simulink model "test20230615"  (R2023b)
settings: Solver=FixedStepAuto  StartTime=0.0  StopTime=20  FixedStep=0.001  RelTol=1e-3
undefined symbols (not defined in the file): DiscIntNeverNeededParam
libraries: simulink x1
settings Model: Creator=DONGGUIYI  LastModifiedBy=dgy92
settings OptimizationCC: ReuseModelBlockBuffer=off

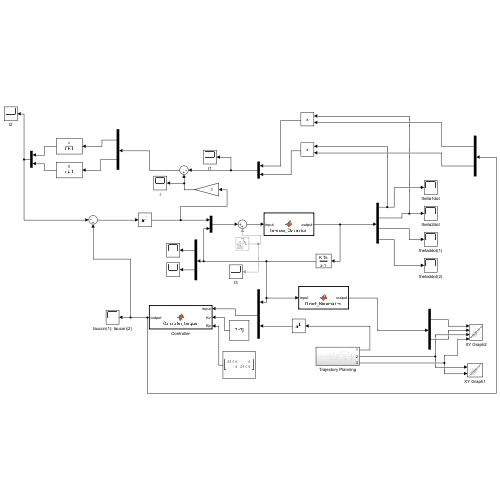
[thumbnail: Simulink's stored preview of the top-level diagram]
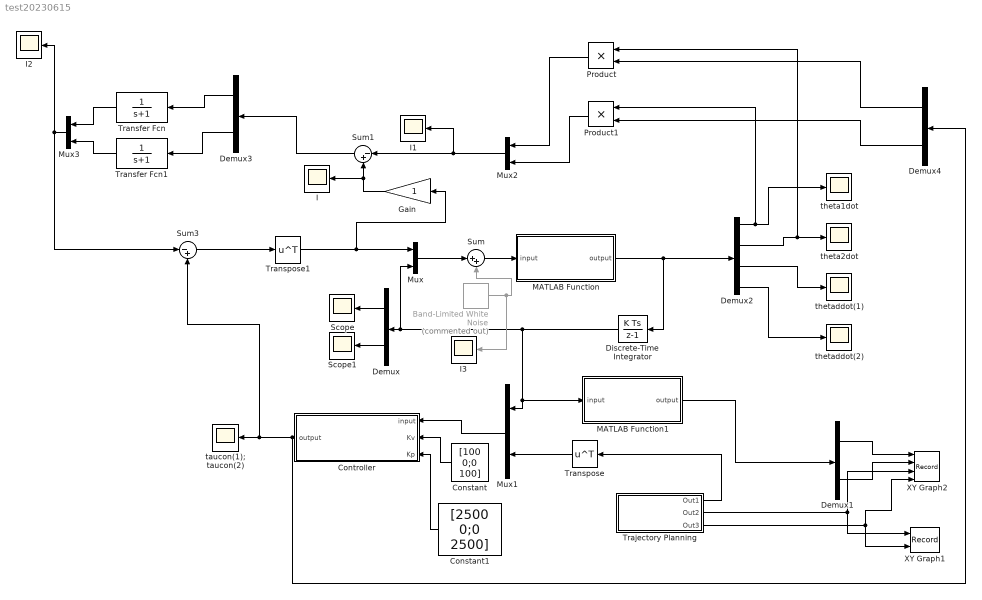
== system test20230615 ==
  Band-Limited White Noise : simulink/Sources/Band-Limited White Noise  Commented=on  Cov=[0.001]  Ts=0.1  seed=[23341]
  Constant : Constant  Value=[100 0;0 100]
  Constant1 : Constant  Value=[2500 0;0 2500]
  Controller : MATLAB Function  Tag=comp_torque  TreatAsAtomicUnit=on
  Demux{,1,3..4} (4 alike) : Demux  Outputs=2
  Demux2 : Demux
  Discrete-Time Integrator : DiscreteIntegrator  SampleTime=-1  ICPrevOutput=DiscIntNeverNeededParam  ICPrevScaledInput=DiscIntNeverNeededParam
  Gain : Gain
  I{,1..3} (4 alike) : Scope
  MATLAB Function : MATLAB Function  TreatAsAtomicUnit=on
  MATLAB Function1 : MATLAB Function  TreatAsAtomicUnit=on
  Mux : Mux  Inputs=[2,4]
  Mux1 : Mux  Inputs=2
  Mux2 : Mux  Inputs=[1,1]
  Mux3 : Mux  Inputs=[1,1]
  Product : Product
  Product1 : Product
  Scope : Scope
  Scope1 : Scope
  Sum : Sum  Inputs=|++
  Sum1 : Sum  Inputs=|-+
  Sum3 : Sum  Inputs=|-+
  Trajectory Planning : Subsystem
  Transfer Fcn : TransferFcn  Denominator=[1 1]
  Transfer Fcn1 : TransferFcn  Denominator=[1 1]
  Transpose : Math  Operator=transpose
  Transpose1 : Math  Operator=transpose
  XY Graph1 : Record  FileSettingsInternal="{\"entries\":[{\"content\":{\"excelSettings\":{\"content\":{},\"type\":\"Streamout.ExcelSettings\"}},\"type\":\"Streamout.FileSettingStorage\",\"uuid\":\"\"}],\"packageUris\":[\"http:\\/\\/schema.mathworks.com\\/mf0\\/streamout_blocks\\/R2020a\"],\"version\":\"1.0\"}"  Layout=[1 1]  SignalsInternal="{\"entries\":[{\"content\":{\"signals\":[{\"content\":{\"blockPath\":[],\"dimensions\":[1,1],\"domain\":\"\",\"lineColor\":\"#77ac30\",\"plots\":[1],\"port\":1,\"sid\":[\"\"],\"signalID\":896,\"signalName\":\"Trajectory Planning:2\"},\"type\":\"RecordBlkView.Signal\",\"uuid\":\"\"},{\"content\":{\"blockPath\":[],\"dimensions\":[1,1],\"domain\":\"\",\"lineColor\":\"#4dbeee\",\"plots\":[1],\"port\":2,\"sid\":[\"\"],\"signalID\":900,\"signalName\":\"Trajectory Planning:3\"},\"type\":\"RecordBlkView.Signal\",\"uuid\":\"\"}]},\"type\":\"RecordBlkView.InputSignals\",\"uuid\":\"\"}],\"packageUris\":[\"http:\\/\\/schema.mathworks.com\\/mf0\\/streamout_blocks\\/R2020a\"],\"version\":\"1.0\"}"  VisualizationBindings="{\"xyplotplugin\":{\"info\":[{\"series\":[{\"bindingParametersList\":[{\"parameter\":\"X-Axis\",\"signalID\":896,\"signalName\":\"Trajectory Planning:2\"},{\"parameter\":\"Y-Axis\",\"signalID\":900,\"signalName\":\"Trajectory Planning:3\"}],\"seriesID\":3912}],\"subplotID\":1}]}}"  CompatibilityTag=XY
  XY Graph2 : Record  FileSettingsInternal="{\"entries\":[{\"content\":{\"excelSettings\":{\"content\":{},\"type\":\"Streamout.ExcelSettings\"}},\"type\":\"Streamout.FileSettingStorage\",\"uuid\":\"\"}],\"packageUris\":[\"http:\\/\\/schema.mathworks.com\\/mf0\\/streamout_blocks\\/R2020a\"],\"version\":\"1.0\"}"  Layout=[1 1]  SignalsInternal="{\"entries\":[{\"content\":{\"signals\":[{\"content\":{\"blockPath\":[],\"dimensions\":[1,1],\"domain\":\"\",\"lineColor\":\"#a2142f\",\"plots\":[1],\"port\":1,\"sid\":[\"\"],\"signalID\":904,\"signalName\":\"Demux1:1\"},\"type\":\"RecordBlkView.Signal\",\"uuid\":\"\"},{\"content\":{\"blockPath\":[],\"dimensions\":[1,1],\"domain\":\"\",\"lineColor\":\"#139fff\",\"plots\":[1],\"port\":2,\"sid\":[\"\"],\"signalID\":908,\"signalName\":\"Demux1:2\"},\"type\":\"RecordBlkView.Signal\",\"uuid\":\"\"},{\"content\":{\"blockPath\":[],\"dimensions\":[1,1],\"domain\":\"\",\"lineColor\":\"#ff6929\",\"plots\":[1],\"port\":3,\"sid\":[\"\"],\"signalID\":912,\"signalName\":\"Trajectory Planning:2\"},\"type\":\"RecordBlkView.Signal\",\"uuid\":\"\"},{\"content\":{\"blockPath\":[],\"dimensions\":[1,1],\"domain\":\"\",\"lineColor\":\"#b746ff\",\"plots\":[1],\"port\":4,\"sid\":[\"\"],\"signalID\":916,\"signalName\":\"Trajectory Planning:3\"},\"type\":\"RecordBlkView.Signal\",\"uuid\":\"\"}]},\"type\":\"RecordBlkView.InputSignals\",\"uuid\":\"\"}],\"packageUris\":[\"http:\\/\\/schema.mathworks.com\\/mf0\\/streamout_blocks\\/R2020a\"],\"version\":\"1.0\"}"  VisualizationBindings="{\"xyplotplugin\":{\"info\":[{\"series\":[{\"bindingParametersList\":[{\"parameter\":\"X-Axis\",\"signalID\":904,\"signalName\":\"Demux1:1\"},{\"parameter\":\"Y-Axis\",\"signalID\":908,\"signalName\":\"Demux1:2\"}],\"seriesID\":2340},{\"bindingParametersList\":[{\"parameter\":\"X-Axis\",\"signalID\":912,\"signalName\":\"Trajectory Planning:2\"},{\"parameter\":\"Y-Axis\",\"signalID\":916,\"signalName\":\"Trajectory Planning:3\"}],\"seriesID\":45430}],\"subplotID\":1}]}}"  CompatibilityTag=XY  st=-1
  taucon(1); taucon(2) : Scope
  theta1dot : Scope
  theta2dot : Scope
  thetaddot(1) : Scope
  thetaddot(2) : Scope
  wires:
  Discrete-Time Integrator/1 -> Mux1/1, MATLAB Function1/1(input), Mux/2, Demux/1
  Demux/2 -> Scope1/1
  Demux/1 -> Scope/1
  MATLAB Function1/1(output) -> Demux1/1
  Demux1/1 -> XY Graph2/1
  Demux1/2 -> XY Graph2/2
  Transpose/1 -> Mux1/2
  Trajectory Planning/1(Out1) -> Transpose/1
  Controller/1(output) -> Demux4/1, Sum3/2, taucon(1); taucon(2)/1
  Mux1/1 -> Controller/1(input)
  Trajectory Planning/2(Out2) -> XY Graph2/3, XY Graph1/1
  Trajectory Planning/3(Out3) -> XY Graph2/4, XY Graph1/2
  Constant/1 -> Controller/2(Kv)
  Constant1/1 -> Controller/3(Kp)
  Demux2/4 -> thetaddot(2)/1
  Demux2/3 -> thetaddot(1)/1
  Demux2/2 -> Product/1, theta2dot/1
  Demux2/1 -> Product1/1, theta1dot/1
  Band-Limited White Noise/1 -> I3/1, Sum/2
  MATLAB Function/1(output) -> Discrete-Time Integrator/1, Demux2/1
  Sum/1 -> MATLAB Function/1(input)
  Mux/1 -> Sum/1
  Mux2/1 -> I1/1, Sum1/1
  Gain/1 -> I/1, Sum1/2
  Sum3/1 -> Transpose1/1
  Transpose1/1 -> Gain/1, Mux/1
  Sum1/1 -> Demux3/1
  Demux3/2 -> Transfer Fcn1/1
  Mux3/1 -> I2/1, Sum3/1
  Demux3/1 -> Transfer Fcn/1
  Transfer Fcn/1 -> Mux3/1
  Transfer Fcn1/1 -> Mux3/2
  Demux4/1 -> Product/2
  Demux4/2 -> Product1/2
  Product/1 -> Mux2/1
  Product1/1 -> Mux2/2

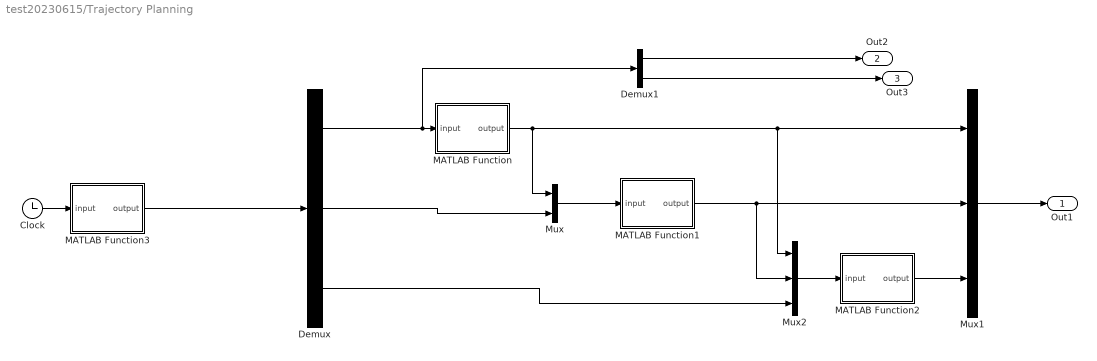
== system test20230615/Trajectory Planning ==
  Clock : Clock
      settings: Decimation=100
  Demux : Demux  Outputs=3
  Demux1 : Demux  Outputs=2
  MATLAB Function : MATLAB Function  TreatAsAtomicUnit=on
  MATLAB Function1 : MATLAB Function  TreatAsAtomicUnit=on
  MATLAB Function2 : MATLAB Function  TreatAsAtomicUnit=on
  MATLAB Function3 : MATLAB Function  TreatAsAtomicUnit=on
  Mux : Mux  Inputs=2
  Mux1 : Mux  Inputs=3
  Mux2 : Mux  Inputs=3
  Out1 : Outport
  Out2 : Outport  Port=2
  Out3 : Outport  Port=3
  wires:
  Demux/3 -> Mux2/3
  Mux1/1 -> Out1/1
  MATLAB Function1/1(output) -> Mux2/2, Mux1/2
  Demux1/2 -> Out3/1
  Mux/1 -> MATLAB Function1/1(input)
  MATLAB Function2/1(output) -> Mux1/3
  Demux/1 -> Demux1/1, MATLAB Function/1(input)
  Mux2/1 -> MATLAB Function2/1(input)
  Demux1/1 -> Out2/1
  Clock/1 -> MATLAB Function3/1(input)
  MATLAB Function/1(output) -> Mux/1, Mux2/1, Mux1/1
  Demux/2 -> Mux/2
  MATLAB Function3/1(output) -> Demux/1

== matlab function test20230615/Trajectory Planning/MATLAB Function ==
  data: input input; output output
function output =angle(input)
x=input(1);
y=input(2);
l1=0.5;
l2=0.5;
a=(x^2+y^2+l1^2+l2^2)^2;
b=2*((x^2+y^2)^2+l1^4+l2^4);
k=sqrt(abs(a-b));
theta1=atan2(y,x)+atan2(k,x^2+y^2+l1^2-l2^2);
theta2=-atan2(k,x^2+y^2-l1^2-l2^2);
output=[theta1;theta2];

== matlab function test20230615/Trajectory Planning/MATLAB Function2 ==
  data: input input; output output
function output =angleddot(input)
theta1=input(1);
theta2=input(2);
theta1dot=input(3);
theta2dot=input(4);
xddot=input(5);
yddot=input(6);
xyddot=[xddot;yddot];
l1=0.5;
l2=0.5;
A=[-l1*sin(theta1)-l2*sin(theta1+theta2) -l2*sin(theta1+theta2)
 l1*cos(theta1)+l2*cos(theta1+theta2) l2*cos(theta1+theta2)];
B11=-l1*cos(theta1)*theta1dot^2-l2*cos(theta1+theta2)*(theta1dot+theta2dot)^2;
B21=-l1*sin(theta1)*theta1dot^2-l2*sin(theta1+theta2)*(theta1dot+theta2dot)^2;
B=[B11;B21];
% to avoid matrix Asingularity
if det(A)<=0.001
 thetaddot=[0.001;0.001];
else
 thetaddot=inv(A)*(xyddot-B);
end;
output=thetaddot;

== matlab function test20230615/Trajectory Planning/MATLAB Function3 ==
  data: input input; output output
function output =xytrajectory(input)
t1=input;
omega = 0.5;
phi=omega*t1;
x=0.2*cos(phi)+0.3;
y=0.2*sin(phi)+0.3;
xdot=-0.2*sin(phi);
ydot=0.2*cos(phi);
xddot=-0.2*cos(phi);
yddot=-0.2*sin(phi);
output=[x;y;xdot;ydot;xddot;yddot];

== matlab function test20230615/MATLAB Function ==
  data: input input; output output
function output =Inverse_Dynamics(input)


m1 = 1.0;
m2 = 1.0;

b1 = 0

b2 = 0

l1 = 0.5

l2 = 0.5

g = 9.81;
torque = [input(1); input(2)];
theta1 = input(3);
theta2 = input(4);
theta1dot = input(5);
theta2dot = input(6);
M11=(m1+m2)*l1^2+m2*l2^2+2*m2*l1*l2*cos(theta2);
M12= m2*l2^2+m2*l1*l2*cos(theta2);
M21=m2*l2^2+m2*l1*l2*cos(theta2);
M22=m2*l2^2;
M = [M11 M12; M21 M22];
V11=-m2*l1*l2*(2*theta1dot*theta2dot+theta1dot^2)*sin(theta2);
V21=m2*l1*l2*theta1dot^2*sin(theta2);
V = [V11;V21];
G11=(m1+m2)*g*l1*cos(theta1)+m2*g*cos(theta1+theta2)*l2;
G21=m2*g*l2*cos(theta1+theta2);
G=[G11;G21];
F = [b1*theta1dot;b2*theta2dot];
thetaddot=inv(M)*(torque-F-V-G);
output=[input(5) input(6) thetaddot(1) thetaddot(2)];

== matlab function test20230615/MATLAB Function1 ==
  data: input input; output output
function output =Direct_Kinematics(input)
theta1=input(1);
theta2=input(2);
l1=0.5; 
l2=0.5;
x=l1*cos(theta1)+l2*cos(theta1+theta2);
y=l1*sin(theta1)+l2*sin(theta1+theta2);
output=[x;y];

== matlab function test20230615/Controller ==
  data: input input; output output; Kv input; Kp input
function output =Controller_torque(input,Kv,Kp)
theta1=input(1);
theta2=input(2);
theta1dot=input(3);
theta2dot=input(4);
thetad1=input(5);
thetad2=input(6);
thetad1dot=input(7);
thetad2dot=input(8);
thetad1ddot=input(9);
thetad2ddot=input(10);
%Kv=[2 0;0 2];
%Kp=[6 0;0 6];
m1 = 1.0;
m2 = 1.0;
b1 = 0;
b2 = 0;
l1 = 0.5;
l2 = 0.5;
g = 9.81;
M11=(m1+m2)*l1^2+m2*l2^2+2*m2*l1*l2*cos(theta2);
M12= m2*l2^2+m2*l1*l2*cos(theta2);
M21=m2*l2^2+m2*l1*l2*cos(theta2);
M22=m2*l2^2;
M = [M11 M12; M21 M22];
V11=-m2*l1*l2*(2*theta1dot*theta2dot+theta1dot^2)*sin(theta2); 
V21=m2*l1*l2*theta1dot^2*sin(theta2);
V = [V11;V21];
G11=(m1+m2)*g*l1*cos(theta1)+m2*g*cos(theta1+theta2)*l2;
G21=m2*g*l2*cos(theta1+theta2);
G=[G11;G21];
F = [b1*theta1dot;b2*theta2dot];
theta = [theta1; theta2];
thetadot = [theta1dot; theta2dot];
thetad = [thetad1; thetad2];
thetaddot = [thetad1dot; thetad2dot];
thetadddot = [thetad1ddot; thetad2ddot];
taucon = M*(thetadddot+Kv*(thetaddot-thetadot)+Kp*(thetad-theta))+V+G+F;
output=[taucon(1); taucon(2)];

== matlab function test20230615/Trajectory Planning/MATLAB Function1 ==
  data: input input; output output
function output =angledot(input)
theta1=input(1);
theta2=input(2);
xdot=input(3);
ydot=input(4);
xydot=[xdot;ydot];
l1=0.5;
l2=0.5;
A=[-l1*sin(theta1)-l2*sin(theta1+theta2) -l2*sin(theta1+theta2)
 l1*cos(theta1)+l2*cos(theta1+theta2) l2*cos(theta1+theta2)];
if det(A)<=0.001
 thetadot=[0;0];
else
 thetadot=inv(A)*xydot;
end;
output=thetadot;
